simulink model "redTrackerTestModel"  (R2013b)
settings: Solver=ode45  StartTime=0.0  StopTime=10.0  RelTol=1e-3
libraries: visionsinks x2, dspvision x1
settings Model: Creator=menkh  LastModifiedBy=menkh

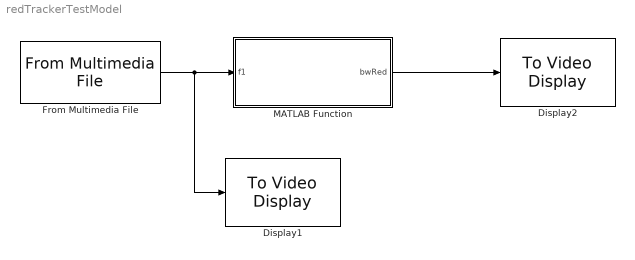
== system redTrackerTestModel ==
  Display1 : visionsinks/To Video Display  inputType=Obsolete  imagePorts=One multidimensional signal  OutputDevice=On-screen video monitor  fullScreen=off  videoWindowX=230  videoWindowY=473  saveWindowSize=off  videoWindowWidth=176  videoWindowHeight=144  dataOrg=Column-major  openAtMdlStart=on  isWindowOpen=off  inputColorFormat=RGB
  Display2 : visionsinks/To Video Display  inputType=Obsolete  imagePorts=One multidimensional signal  OutputDevice=On-screen video monitor  fullScreen=off  videoWindowX=170  videoWindowY=354  saveWindowSize=off  videoWindowWidth=176  videoWindowHeight=144  dataOrg=Column-major  openAtMdlStart=on  isWindowOpen=on  inputColorFormat=RGB
  From Multimedia File : dspvision/From Multimedia File  inputFilename=natickTrial1.mp4  loop=on  numPlays=inf  outputStreams=Video only  videoDataType=uint8  audioDataType=int16  inheritSampleTime=on  userDefinedSampleTime=1/30  noAudioOutput=off  isIntensityVideo=off  fourcc=RGB  colorVideoFormat=One multidimensional signal  outputEOF=off  dataOrg=Column-major  audioFrameSize=1024  computeAudioFrameSize=off  outSamplingMode=Sample based
  MATLAB Function : MATLAB Function  TreatAsAtomicUnit=on
  wires:
  From Multimedia File/1 -> MATLAB Function/1(f1), Display1/1
  MATLAB Function/1(bwRed) -> Display2/1

== matlab function redTrackerTestModel/MATLAB Function ==
  data: f1 input; bwRed output
function bwRed = redTracker(f1)
%#codegen

greyThreshold = 30;
rgThreshold = 20;
gbThreshold = 20;
rbThreshold = 20;

vidHeight = 144;
vidWidth = 176;

%RG channel
frg = f1(:, :, 1 : 2);
%GB channel
fgb = f1(:, :, 2 : 3);
%RB channel
frb = zeros(vidHeight, vidWidth, 2);
frb(:, :, 1) = f1(:, :, 1);
frb(:, :, 2) = f1(:, :, 3);

%null indexes
greynull = max(f1, [], 3) - min(f1, [], 3) < greyThreshold;
rgnull = max(frg, [], 3) - min(frg, [], 3) < rgThreshold;
gbnull = max(fgb, [], 3) - min(fgb, [], 3) < gbThreshold;
rbnull = max(frb, [], 3) - min(frb, [], 3) < rbThreshold;

%dominant indexes (GB null)
rdom = (max(f1, [], 3) - f1(:, :, 1)) < 1;


% f1_f = zeros(vidHeight, vidWidth, 2);
%red----------------------------
% fcred = f1(:, :, 1);
fcred = zeros(vidHeight, vidWidth);
fcred(rdom) = 255;

%strip greyscale
fcred(greynull) = 0;

%strip RG
fcred(rgnull) = 0;

%strip GB
fcred(gbnull & ~rdom) = 0;

%strip RB
fcred(rbnull) = 0;

%filter for R dominance
fcred(~rdom) = 0;

%reconstruct image
% f1_f(:, :, 1) = fcred;
bwRed = fcred;
